simulink library "iPendulumLibrary"  (R2016b)
settings: Solver=ode45  StartTime=0.0  StopTime=10.0  RelTol=1e-3  EnableMultiTasking=on
undefined symbols (not defined in the file): C, dphi0, dtheta0, dx0, g, I, Iw, M, theta0, u_max
libraries: iPendulumLibrary x2
settings Model: Creator=Christian  LastModifiedBy=Chris
settings DataIOCC: LimitDataPoints=on  SaveFormat=Array
settings OptimizationCC: LifeSpan=inf
settings DebuggingCC: AllowSymbolicDim=off  SFUnexpectedBacktrackingDiag=warning  SFNoUnconditionalDefaultTransitionDiag=warning  SFExecutionAtInitializationDiag=none
settings HardwareCC: ProdBitPerPointer=32  ProdBitPerSizeT=32  ProdBitPerPtrDiffT=32  ProdLargestAtomicFloat=None  ProdIntDivRoundTo=Undefined  ProdEndianess=Unspecified  ProdWordSize=32  ProdHWDeviceType=32-bit Generic
settings ModelReferenceCC: PropagateSignalLabelsOutOfModel=off
settings GRTTargetCC: TargetLangStandard=C89/C90 (ANSI)  GeneratePreprocessorConditionals=Disable all
settings ConfigComp: CovMetricSettings=dw  CovHtmlReporting=on  CovSaveCumulativeToWorkspaceVar=on  CovSaveSingleToWorkspaceVar=on  CovExternalEMLEnable=off

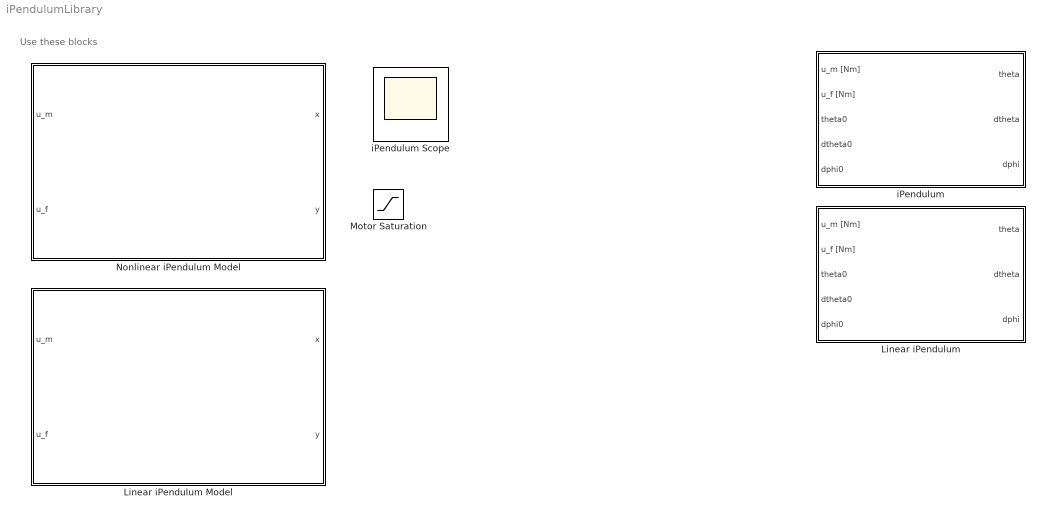
== system iPendulumLibrary ==
  note: Use these blocks
  Linear iPendulum : Subsystem
      mask Display:
      | plot([-4 0 4 -4],[4 0 4 4])
      | patch(0+[sin(0), sin(pi* 1/12), sin(pi* 2/12), sin(pi* 3/12), sin(pi* 4/12), sin(pi* 5/12), sin(pi* 6/12), sin(pi* 7/12), sin(pi* 8/12), sin(pi* 9/12), sin(pi* 10/12), sin(pi* 11/12), sin(pi* 12/12), sin(pi* 13/12), sin(pi* 14/12), sin(pi* 15/12), sin(pi* 16/12), sin(pi* 17/12), sin(pi* 18/12), sin(pi* 19/12), sin(pi* 20/12), sin(pi* 21/12), sin(pi* 22/12), sin(pi* 23/12)]*1,2+[cos(0), cos(pi* 1/12), cos(pi* 2/12), cos(pi* 3/12), cos(pi* 4/12), cos(pi* 5/12), cos(pi* 6/12), cos(pi* 7/12), cos(pi* 8/12), cos(pi* 9/12), cos(pi* 10/12), cos(pi* 11/12), cos(pi* 12/12), cos(pi* 13/12), cos(pi* 14/12), cos(pi* 15/12), cos(pi* 16/12), cos(pi* 17/12), cos(pi* 18/12), cos(pi* 19/12), cos(pi* 20/12), cos(pi* 21/12), cos(pi* 22/12), cos(pi* 23/12)]*1)
      | text(-7, 7, '')
      | text( 7, 7, '')
      | text( 0, -2, '')
      | text(-3, 5, 'Linearized\n Model (upright)')
      | port_label('output', 1, 'theta [rad]')
      | port_label('output', 2, 'dtheta [rad/s]')
      | port_label('output', 3, 'dphi [rad/s]')
      | port_label('input',  1, 'u_m [Nm]')
      | port_label('input',  2, 'u_f [Nm]')
      | port_label('input',  3, 'theta0 [rad]')
      | port_label('input',  4, 'dtheta0 [rad/s]')
      | port_label('input',  5, 'dphi0 [rad/s]')
  Linear iPendulum Model : Subsystem
      mask Display:
      | plot([-4 0 4 -4],[4 0 4 4])
      | patch(0+[sin(0), sin(pi* 1/12), sin(pi* 2/12), sin(pi* 3/12), sin(pi* 4/12), sin(pi* 5/12), sin(pi* 6/12), sin(pi* 7/12), sin(pi* 8/12), sin(pi* 9/12), sin(pi* 10/12), sin(pi* 11/12), sin(pi* 12/12), sin(pi* 13/12), sin(pi* 14/12), sin(pi* 15/12), sin(pi* 16/12), sin(pi* 17/12), sin(pi* 18/12), sin(pi* 19/12), sin(pi* 20/12), sin(pi* 21/12), sin(pi* 22/12), sin(pi* 23/12)]*1,2+[cos(0), cos(pi* 1/12), cos(pi* 2/12), cos(pi* 3/12), cos(pi* 4/12), cos(pi* 5/12), cos(pi* 6/12), cos(pi* 7/12), cos(pi* 8/12), cos(pi* 9/12), cos(pi* 10/12), cos(pi* 11/12), cos(pi* 12/12), cos(pi* 13/12), cos(pi* 14/12), cos(pi* 15/12), cos(pi* 16/12), cos(pi* 17/12), cos(pi* 18/12), cos(pi* 19/12), cos(pi* 20/12), cos(pi* 21/12), cos(pi* 22/12), cos(pi* 23/12)]*1)
      | text(-7, 7, '')
      | text( 7, 7, '')
      | text( 0, -2, '')
      | text(-3, 5, 'Linearized\n Model')
      | port_label('output', 1, 'x = [theta, dtheta, dphi]') %
      | port_label('output', 2, 'y = [theta, dphi]') %
      | port_label('input',  1, 'u_m [Nm]')
      | port_label('input',  2, 'u_f [Nm]')
  Motor Saturation : Saturate  UpperLimit=u_max  LowerLimit=-u_max
  Nonlinear iPendulum Model : Subsystem
      mask Display:
      | plot([-4 0 4 -4],[4 0 4 4])
      | patch(0+[sin(0), sin(pi* 1/12), sin(pi* 2/12), sin(pi* 3/12), sin(pi* 4/12), sin(pi* 5/12), sin(pi* 6/12), sin(pi* 7/12), sin(pi* 8/12), sin(pi* 9/12), sin(pi* 10/12), sin(pi* 11/12), sin(pi* 12/12), sin(pi* 13/12), sin(pi* 14/12), sin(pi* 15/12), sin(pi* 16/12), sin(pi* 17/12), sin(pi* 18/12), sin(pi* 19/12), sin(pi* 20/12), sin(pi* 21/12), sin(pi* 22/12), sin(pi* 23/12)]*1,2+[cos(0), cos(pi* 1/12), cos(pi* 2/12), cos(pi* 3/12), cos(pi* 4/12), cos(pi* 5/12), cos(pi* 6/12), cos(pi* 7/12), cos(pi* 8/12), cos(pi* 9/12), cos(pi* 10/12), cos(pi* 11/12), cos(pi* 12/12), cos(pi* 13/12), cos(pi* 14/12), cos(pi* 15/12), cos(pi* 16/12), cos(pi* 17/12), cos(pi* 18/12), cos(pi* 19/12), cos(pi* 20/12), cos(pi* 21/12), cos(pi* 22/12), cos(pi* 23/12)]*1)
      | text(-7, 7, '')
      | text( 7, 7, '')
      | text( 0, -2, '')
      | text(-3, 5, 'Nonlinear\n Model')
      | port_label('output', 1, 'x = [theta, dtheta, dphi]') %
      | port_label('output', 2, 'y = [theta, dphi]') %
      | port_label('input',  1, 'u_m [Nm]')
      | port_label('input',  2, 'u_f [Nm]')
  iPendulum : Subsystem
      mask Display:
      | plot([-4 0 4 -4],[4 0 4 4])
      | patch(0+[sin(0), sin(pi* 1/12), sin(pi* 2/12), sin(pi* 3/12), sin(pi* 4/12), sin(pi* 5/12), sin(pi* 6/12), sin(pi* 7/12), sin(pi* 8/12), sin(pi* 9/12), sin(pi* 10/12), sin(pi* 11/12), sin(pi* 12/12), sin(pi* 13/12), sin(pi* 14/12), sin(pi* 15/12), sin(pi* 16/12), sin(pi* 17/12), sin(pi* 18/12), sin(pi* 19/12), sin(pi* 20/12), sin(pi* 21/12), sin(pi* 22/12), sin(pi* 23/12)]*1,2+[cos(0), cos(pi* 1/12), cos(pi* 2/12), cos(pi* 3/12), cos(pi* 4/12), cos(pi* 5/12), cos(pi* 6/12), cos(pi* 7/12), cos(pi* 8/12), cos(pi* 9/12), cos(pi* 10/12), cos(pi* 11/12), cos(pi* 12/12), cos(pi* 13/12), cos(pi* 14/12), cos(pi* 15/12), cos(pi* 16/12), cos(pi* 17/12), cos(pi* 18/12), cos(pi* 19/12), cos(pi* 20/12), cos(pi* 21/12), cos(pi* 22/12), cos(pi* 23/12)]*1)
      | text(-7, 7, '')
      | text( 7, 7, '')
      | text( 0, -2, '')
      | text(-3, 5, 'Nonlinear\n Model')
      | port_label('output', 1, 'theta [rad]')
      | port_label('output', 2, 'dtheta [rad/s]')
      | port_label('output', 3, 'dphi [rad/s]')
      | port_label('input',  1, 'u_m [Nm]')
      | port_label('input',  2, 'u_f [Nm]')
      | port_label('input',  3, 'theta0 [rad]')
      | port_label('input',  4, 'dtheta0 [rad/s]')
      | port_label('input',  5, 'dphi0 [rad/s]')
  iPendulum Scope : Scope  NumInputPorts=3

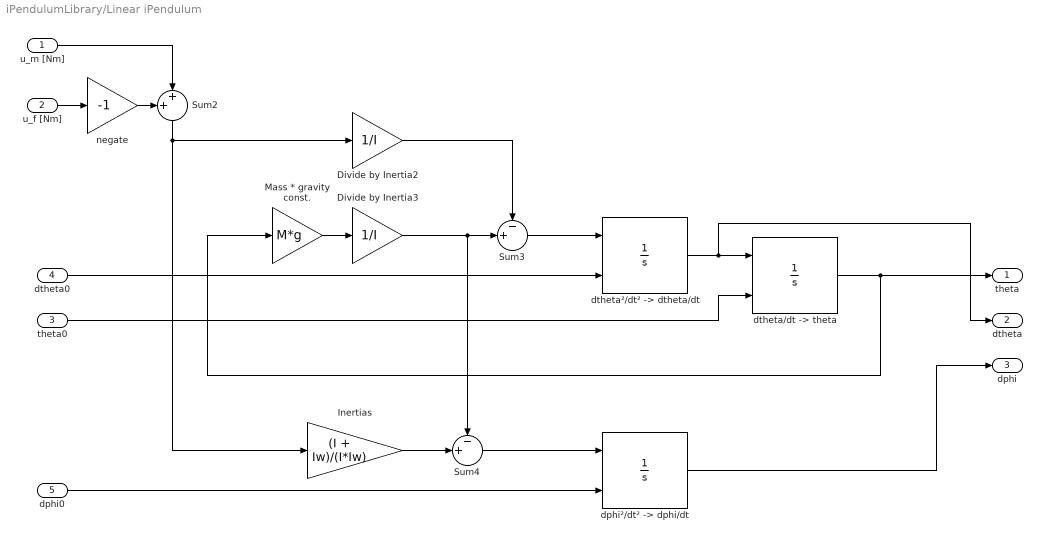
== system iPendulumLibrary/Linear iPendulum ==
  u_m [Nm] : Inport
  u_f [Nm] : Inport  Port=2
  theta0 : Inport  Port=3
  dtheta0 : Inport  Port=4
  dphi0 : Inport  Port=5
  Divide by Inertia2 : Gain  Gain=1/I
  Divide by Inertia3 : Gain  Gain=1/I
  Inertias : Gain  Gain=(I + Iw)/(I*Iw)
  Mass * gravity const. : Gain  Gain=M*g
  Sum2 : Sum  Inputs=++|
  Sum3 : Sum  Inputs=-+|
  Sum4 : Sum  Inputs=-+|
  "dphi²/dt² -> dphi/dt" : Integrator  InitialConditionSource=external  InitialCondition=[dx0, dphi0]
  "dtheta/dt -> theta" : Integrator  InitialConditionSource=external  InitialCondition=[dx0, dphi0]
  "dtheta²/dt² -> dtheta/dt" : Integrator  InitialConditionSource=external  InitialCondition=[dx0, dphi0]
  negate : Gain  Gain=-1
  theta : Outport
  dtheta : Outport  Port=2
  dphi : Outport  Port=3
  wires:
  Sum4/1 -> "dphi²/dt² -> dphi/dt"/1
  Sum2/1 -> Divide by Inertia2/1, Inertias/1
  Inertias/1 -> Sum4/2
  Divide by Inertia3/1 -> Sum3/2, Sum4/1
  Divide by Inertia2/1 -> Sum3/1
  "dphi²/dt² -> dphi/dt"/1 -> dphi/1
  dphi0/1 -> "dphi²/dt² -> dphi/dt"/2
  "dtheta/dt -> theta"/1 -> Mass * gravity const./1, theta/1
  theta0/1 -> "dtheta/dt -> theta"/2
  "dtheta²/dt² -> dtheta/dt"/1 -> "dtheta/dt -> theta"/1, dtheta/1
  Sum3/1 -> "dtheta²/dt² -> dtheta/dt"/1
  Mass * gravity const./1 -> Divide by Inertia3/1
  negate/1 -> Sum2/1
  u_f [Nm]/1 -> negate/1
  u_m [Nm]/1 -> Sum2/2
  dtheta0/1 -> "dtheta²/dt² -> dtheta/dt"/2

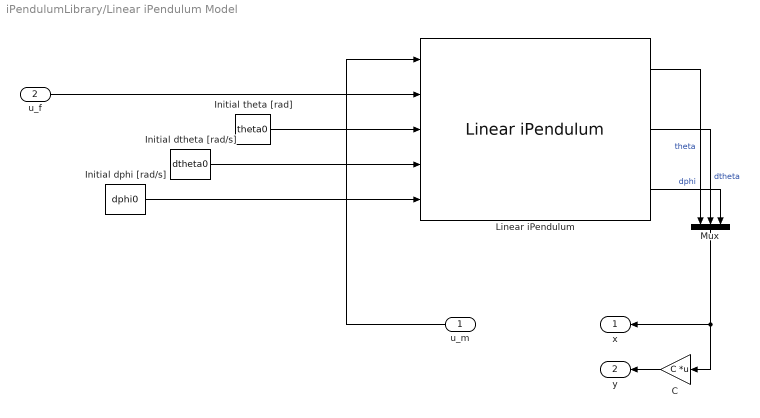
== system iPendulumLibrary/Linear iPendulum Model ==
  u_m : Inport
  u_f : Inport  Port=2
  C : Gain  Gain=C  Multiplication=Matrix(K*u) (u vector)
  Initial dphi [rad/s] : Constant  Value=dphi0
  Initial dtheta [rad/s] : Constant  Value=dtheta0
  Initial theta [rad] : Constant  Value=theta0
  Linear iPendulum : iPendulumLibrary/Linear iPendulum  SystemSampleTime=-1
  Mux : Mux  Inputs=3
  x : Outport
  y : Outport  Port=2
  wires:
  C/1 -> y/1
  Linear iPendulum/1 -> Mux/1  "theta"
  u_m/1 -> Linear iPendulum/1
  Mux/1 -> x/1, C/1
  u_f/1 -> Linear iPendulum/2
  Initial dtheta [rad/s]/1 -> Linear iPendulum/4
  Initial dphi [rad/s]/1 -> Linear iPendulum/5
  Initial theta [rad]/1 -> Linear iPendulum/3
  Linear iPendulum/2 -> Mux/2  "dtheta"
  Linear iPendulum/3 -> Mux/3  "dphi"

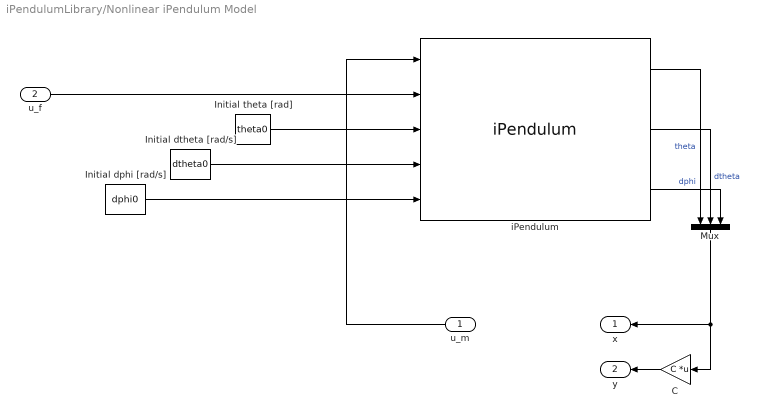
== system iPendulumLibrary/Nonlinear iPendulum Model ==
  u_m : Inport
  u_f : Inport  Port=2
  C : Gain  Gain=C  Multiplication=Matrix(K*u) (u vector)
  Initial dphi [rad/s] : Constant  Value=dphi0
  Initial dtheta [rad/s] : Constant  Value=dtheta0
  Initial theta [rad] : Constant  Value=theta0
  Mux : Mux  Inputs=3
  iPendulum : iPendulumLibrary/iPendulum  SystemSampleTime=-1
  x : Outport
  y : Outport  Port=2
  wires:
  iPendulum/3 -> Mux/3  "dphi"
  iPendulum/2 -> Mux/2  "dtheta"
  Initial theta [rad]/1 -> iPendulum/3
  Initial dphi [rad/s]/1 -> iPendulum/5
  Initial dtheta [rad/s]/1 -> iPendulum/4
  u_f/1 -> iPendulum/2
  Mux/1 -> C/1, x/1
  u_m/1 -> iPendulum/1
  iPendulum/1 -> Mux/1  "theta"
  C/1 -> y/1

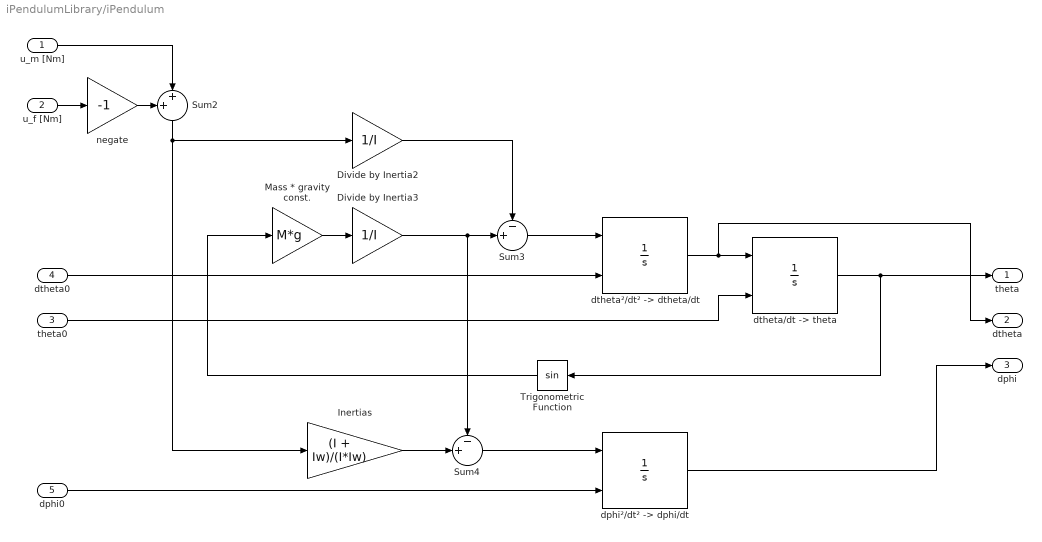
== system iPendulumLibrary/iPendulum ==
  u_m [Nm] : Inport
  u_f [Nm] : Inport  Port=2
  theta0 : Inport  Port=3
  dtheta0 : Inport  Port=4
  dphi0 : Inport  Port=5
  Divide by Inertia2 : Gain  Gain=1/I
  Divide by Inertia3 : Gain  Gain=1/I
  Inertias : Gain  Gain=(I + Iw)/(I*Iw)
  Mass * gravity const. : Gain  Gain=M*g
  Sum2 : Sum  Inputs=++|
  Sum3 : Sum  Inputs=-+|
  Sum4 : Sum  Inputs=-+|
  Trigonometric Function : Trigonometry
  "dphi²/dt² -> dphi/dt" : Integrator  InitialConditionSource=external  InitialCondition=[dx0, dphi0]
  "dtheta/dt -> theta" : Integrator  InitialConditionSource=external  InitialCondition=[dx0, dphi0]
  "dtheta²/dt² -> dtheta/dt" : Integrator  InitialConditionSource=external  InitialCondition=[dx0, dphi0]
  negate : Gain  Gain=-1
  theta : Outport
  dtheta : Outport  Port=2
  dphi : Outport  Port=3
  wires:
  dtheta0/1 -> "dtheta²/dt² -> dtheta/dt"/2
  u_m [Nm]/1 -> Sum2/2
  u_f [Nm]/1 -> negate/1
  negate/1 -> Sum2/1
  Mass * gravity const./1 -> Divide by Inertia3/1
  Sum3/1 -> "dtheta²/dt² -> dtheta/dt"/1
  "dtheta²/dt² -> dtheta/dt"/1 -> dtheta/1, "dtheta/dt -> theta"/1
  theta0/1 -> "dtheta/dt -> theta"/2
  "dtheta/dt -> theta"/1 -> theta/1, Trigonometric Function/1
  Trigonometric Function/1 -> Mass * gravity const./1
  dphi0/1 -> "dphi²/dt² -> dphi/dt"/2
  "dphi²/dt² -> dphi/dt"/1 -> dphi/1
  Divide by Inertia2/1 -> Sum3/1
  Divide by Inertia3/1 -> Sum4/1, Sum3/2
  Inertias/1 -> Sum4/2
  Sum2/1 -> Inertias/1, Divide by Inertia2/1
  Sum4/1 -> "dphi²/dt² -> dphi/dt"/1
